simulink model "victim_direction"  (Simulink 8.7)
settings: Solver=FixedStepAuto  StartTime=0.0  StopTime=inf  FixedStep=0.01  RelTol=1e-3
settings Model: Creator=maximilian  LastModifiedBy=eispin
settings DataIOCC: LimitDataPoints=off  SaveFormat=Dataset
settings DebuggingCC: UnderspecifiedInitializationDetection=Simplified  MergeDetectMultiDrivingBlocksExec=error
settings HardwareCC: ProdBitPerPointer=64  ProdLargestAtomicFloat=Float  ProdIntDivRoundTo=Zero  ProdEndianess=LittleEndian  ProdWordSize=64  ProdHWDeviceType=Intel->x86-64 (Windows64)
settings ModelReferenceCC: PropagateSignalLabelsOutOfModel=on
settings ConfigComp: CovModelRefEnable=off

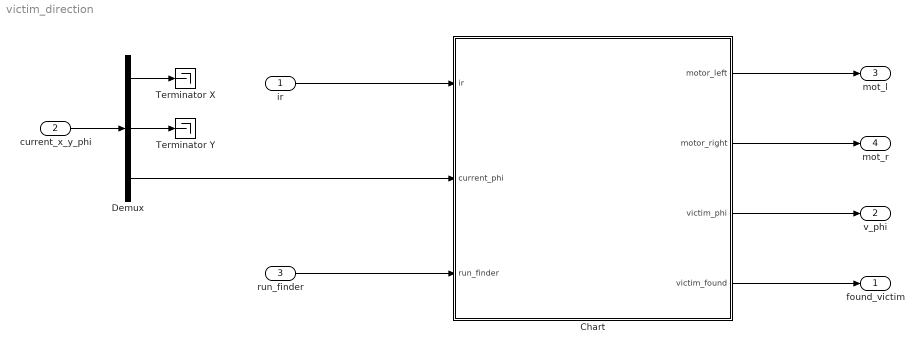
== system victim_direction ==
  ir : Inport  OutDataTypeStr=boolean  PortDimensions=[6]
  current_x_y_phi : Inport  Port=2  PortDimensions=[3]
  run_finder : Inport  Port=3
  Chart : Stateflow chart  TreatAsAtomicUnit=on
  Demux : Demux  Outputs=3
  Terminator X : Terminator
  Terminator Y : Terminator
  found_victim : Outport
  v_phi : Outport  Port=2
  mot_l : Outport  Port=3
  mot_r : Outport  Port=4
  wires:
  Chart/1(motor_left) -> mot_l/1
  Chart/2(motor_right) -> mot_r/1
  Chart/3(victim_phi) -> v_phi/1
  Chart/4(victim_found) -> found_victim/1
  ir/1 -> Chart/1(ir)
  run_finder/1 -> Chart/3(run_finder)
  current_x_y_phi/1 -> Demux/1
  Demux/3 -> Chart/2(current_phi)
  Demux/1 -> Terminator X/1
  Demux/2 -> Terminator Y/1

== stateflow chart Chart ==
  state On
    state Start
      entry:
      % Precondition: At least one sensor
      % deos not detect an IR signal.
      victim_found = 0;
      sensor = -1;
      for i = 1:6
      if ir(i) == 0
      sensor = i;
      end
      end
      assert(ir(sensor) == 0);
      motor_left = -1;
      motor_right = 1;
      initial_phi = current_phi;
    state FoundStart
      entry:
      bound1 = current_phi;
    state FoundEnd
      entry:
      victim_phi = determine_victim_phi(bound1, current_phi, sensor);
    state Done
      entry:
      victim_found = 1;
      motor_right = 0;
      motor_left = 0;
    (default) -> Start
    Start -> FoundStart : [ir(sensor) == 1]
    FoundStart -> FoundEnd : [ir(sensor) == 0]
    FoundEnd -> Done : [abs(current_phi - initial_phi) < 4*pi/180]
  state Off
    entry:
    motor_left = 0;
    motor_right = 0;
  (default) -> Off
  On -> Off : [run_finder == 0]
      | {victim_found = 0;}
  Off -> On : [run_finder == 1]
  data: motor_left output double; ir input double; current_phi input double; motor_right output double; victim_phi output double; victim_found output double; bound1 local double; i local double; sensor local double; run_finder input double; initial_phi local double
